simulink model "ProjectOverview"  (R2019b)
settings: Solver=VariableStepAuto  StartTime=0.0  StopTime=10.0  RelTol=1e-3
settings Model: Creator=lvkoala  LastModifiedBy=lvkoala

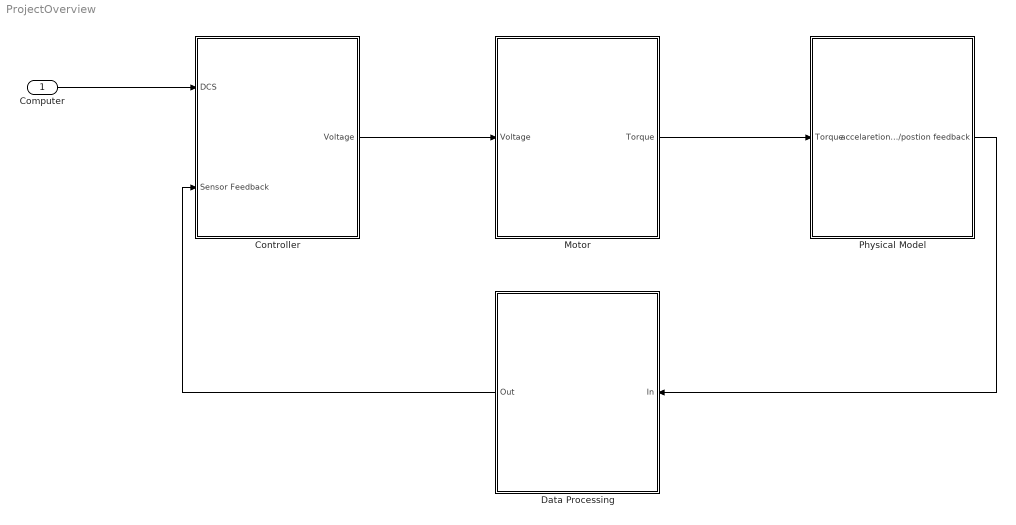
== system ProjectOverview ==
  Computer : Inport
  Controller : Subsystem
  Data Processing : Subsystem
  Motor : Subsystem
  Physical Model : Subsystem
  wires:
  Controller/1(Voltage) -> Motor/1(Voltage)
  Motor/1(Torque) -> Physical Model/1(Torque)
  Computer/1 -> Controller/1(DCS)
  Data Processing/1(Out) -> Controller/2(Sensor Feedback)
  Physical Model/1(accelaretion/postion feedback) -> Data Processing/1(In)

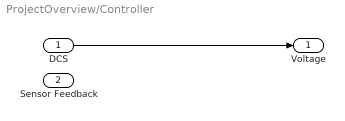
== system ProjectOverview/Controller ==
  DCS : Inport
  Sensor Feedback : Inport  Port=2
  Voltage : Outport
  wires:
  DCS/1 -> Voltage/1

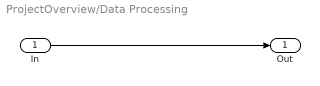
== system ProjectOverview/Data Processing ==
  In : Inport
  Out : Outport
  wires:
  In/1 -> Out/1

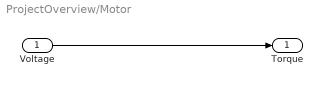
== system ProjectOverview/Motor ==
  Voltage : Inport
  Torque : Outport
  wires:
  Voltage/1 -> Torque/1

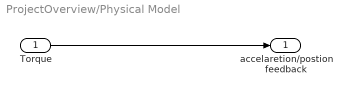
== system ProjectOverview/Physical Model ==
  Torque : Inport
  accelaretion/postion feedback : Outport
  wires:
  Torque/1 -> accelaretion/postion feedback/1
